simulink library "powerlib_models"  (Simulink 6.0)
settings: Solver=ode45  SolverMode=SingleTasking  StartTime=0.0  StopTime=10.0  RelTol=1e-3
values from neighbouring files (symbols this model uses):
  Ts = get(handles.edit1,'string')    [powergui.m]
undefined symbols (not defined in the file or in its folder): A, a0, a1, a2, a3, a4, a5, Ac, Amplitude, Amplitudes, B, BaseCurrent, BaseFlux, Bc, C, Capacitance, Cc, Columns, ConnectionType, Cs, ctrl, current, Current, damp, Dc, Dd, DiscIntNeverNeededParam, dref, dwo, exc, excAxis, F, Flux, fnom, Frequency, FreqVps, Gain1, gate, GH, GHd, GI, GId, GL, GLd, H, HarmonicGeneration, HT, hyd, I1_init, ib, ib2, Id1o, Inductance, InitialFlux, InitialSlope, io, Iq1o, isfinite, j, J ... (+138)
libraries: powerlib_models x32, powerlib_extras x4
(part 3 of 11)

== system powerlib_models/Continuous/diode (logical) ==
  v : Inport  Port=1  LatchInput=off
  0 {1..4} (4 alike) : Constant  Value=0
  Break Alg. Loop : Subsystem  mask{Nsw=1}
      mask prompts: Nsw "number of switches"
  Constant : Constant  Value=zeros(Nsw,1)
  Data Type  Conversion1 : DataTypeConversion  OutDataTypeMode=boolean  SaturateOnIntegerOverflow=on  RndMeth=Zero
  Data Type  Conversion2 : DataTypeConversion  OutDataTypeMode=boolean  SaturateOnIntegerOverflow=on  RndMeth=Zero
  Data Type  Conversion3 : DataTypeConversion  OutDataTypeMode=boolean  SaturateOnIntegerOverflow=on  RndMeth=Zero
  Gain : Gain  Gain=1./Rsw  SaturateOnIntegerOverflow=on
  Mux : Mux  Inputs=2
  Saturation : Saturate  UpperLimit=inf  LowerLimit=0
  Sum : Sum  Inputs=|++  SaturateOnIntegerOverflow=on  InputSameDT=on
  Switch : Switch  Threshold=0.5  InputSameDT=on
  b5 : RelationalOperator  Operator=>  InputSameDT=on
  b6 : RelationalOperator  Operator=>  InputSameDT=on
  b7 : RelationalOperator  Operator===  InputSameDT=on
  or2 : Logic  Operator=OR
  or3 : Logic
  vf : Constant  Value=Vf
  i : Outport  InitialOutput=0
  status : Outport  Port=2  InitialOutput=0
  m : Outport  Port=3  InitialOutput=0
  Vf : Outport  Port=4  InitialOutput=0
  wires:
  0 3/1 -> b7/2
  0 2/1 -> b6/2
  v/1 -> b6/1, Gain/1, Sum/1  "Diode voltage"
  Mux/1 -> m/1  "measurement signals"
  b6/1 -> Data Type  Conversion2/1  "Voltage > 0"
  or3/1 -> or2/2
  or2/1 -> Break Alg. Loop/1(In1)
  Break Alg. Loop/1(Out1) -> status/1, Switch/2  "status"
  0 4/1 -> b5/2
  b5/1 -> Data Type  Conversion1/1  "Current > 0"
  Constant/1 -> i/1
  Sum/1 -> Mux/2  "V = Vak + Vf"
  vf/1 -> Sum/2, Vf/1
  b7/1 -> Data Type  Conversion3/1  "Current = 0"
  Data Type  Conversion1/1 -> or2/1
  Data Type  Conversion2/1 -> or3/1
  Data Type  Conversion3/1 -> or3/2
  Switch/1 -> Saturation/1
  0 1/1 -> Switch/3
  Saturation/1 -> Mux/1, b7/1, b5/1  "Diode current"
  Gain/1 -> Switch/1  "Diode current"

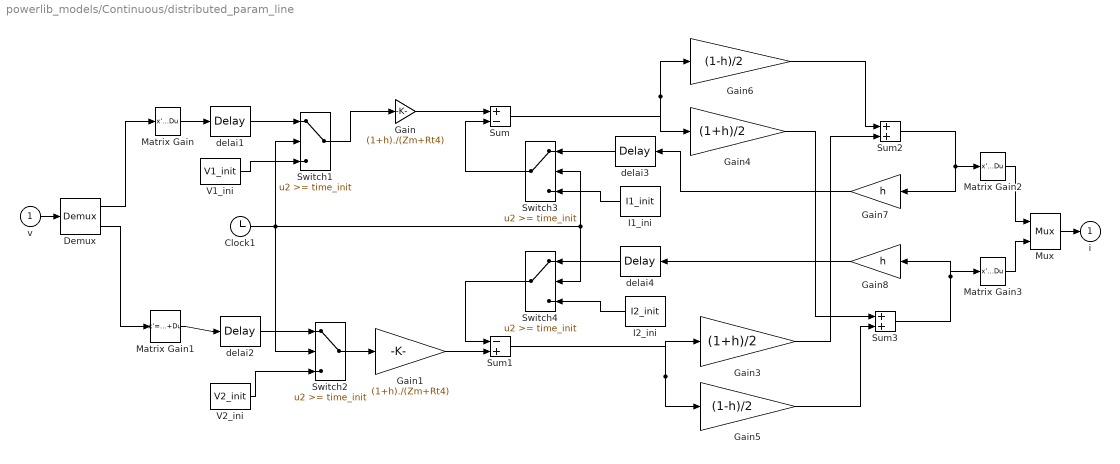
== system powerlib_models/Continuous/distributed_param_line ==
  v : Inport  Port=1  LatchInput=off
  Clock1 : Clock
      settings: Decimation=10
  Demux : Demux  Outputs=[nphase,nphase]
  Gain : Gain  Gain=(1+h)./(Zm+Rt4)  SaturateOnIntegerOverflow=on
  Gain1 : Gain  Gain=(1+h)./(Zm+Rt4)  SaturateOnIntegerOverflow=on
  Gain3 : Gain  Gain=(1+h)/2  SaturateOnIntegerOverflow=on
  Gain4 : Gain  Gain=(1+h)/2  SaturateOnIntegerOverflow=on
  Gain5 : Gain  Gain=(1-h)/2  SaturateOnIntegerOverflow=on
  Gain6 : Gain  Gain=(1-h)/2  SaturateOnIntegerOverflow=on
  Gain7 : Gain  Orientation=left  Gain=h  SaturateOnIntegerOverflow=on
  Gain8 : Gain  Orientation=left  Gain=h  SaturateOnIntegerOverflow=on
  I1_ini : FromWorkspace  Orientation=left  VariableName=I1_init  SampleTime=0
  I2_ini : FromWorkspace  Orientation=left  VariableName=I2_init  SampleTime=0
  Matrix Gain : StateSpace  A=[]  B=[]  C=[]  D=K  mask(Matrix Gain){@1=Ti'}
      mask prompts: @1 "Gain matrix:"
      mask help: Matrix Gain.
      mask init:
      | K = @1;
      mask Help: Multiplies input vector by entered matrix to produce output vector (y=Au).
      mask Display: disp('K')
  Matrix Gain1 : StateSpace  A=[]  B=[]  C=[]  D=K  mask(Matrix Gain){@1=Ti'}
      mask prompts: @1 "Gain matrix:"
      mask help: Matrix Gain.
      mask init:
      | K = @1;
      mask Help: Multiplies input vector by entered matrix to produce output vector (y=Au).
      mask Display: disp('K')
  Matrix Gain2 : StateSpace  A=[]  B=[]  C=[]  D=K  mask(Matrix Gain){@1=Ti}
      mask prompts: @1 "Gain matrix:"
      mask help: Matrix Gain.
      mask init:
      | K = @1;
      mask Help: Multiplies input vector by entered matrix to produce output vector (y=Au).
      mask Display: disp('K')
  Matrix Gain3 : StateSpace  A=[]  B=[]  C=[]  D=K  mask(Matrix Gain){@1=Ti}
      mask prompts: @1 "Gain matrix:"
      mask help: Matrix Gain.
      mask init:
      | K = @1;
      mask Help: Multiplies input vector by entered matrix to produce output vector (y=Au).
      mask Display: disp('K')
  Mux : Mux  Inputs=[nphase,nphase]
  Sum : Sum  Inputs=+-  SaturateOnIntegerOverflow=on  InputSameDT=on
  Sum1 : Sum  Inputs=-+  SaturateOnIntegerOverflow=on  InputSameDT=on
  Sum2 : Sum  SaturateOnIntegerOverflow=on  InputSameDT=on
  Sum3 : Sum  SaturateOnIntegerOverflow=on  InputSameDT=on
  Switch1 : Switch  Threshold=time_init  InputSameDT=on
  Switch2 : Switch  Threshold=time_init  InputSameDT=on
  Switch3 : Switch  Orientation=left  Threshold=time_init  InputSameDT=on
  Switch4 : Switch  Orientation=left  Threshold=time_init  InputSameDT=on
  V1_ini : FromWorkspace  VariableName=V1_init  SampleTime=0
  V2_ini : FromWorkspace  VariableName=V2_init  SampleTime=0
  delai1 : TransportDelay  DelayTime=to
  delai2 : TransportDelay  DelayTime=to
  delai3 : TransportDelay  Orientation=left  DelayTime=to
  delai4 : TransportDelay  Orientation=left  DelayTime=to
  i : Outport  InitialOutput=0
  wires:
  Matrix Gain2/1 -> Mux/1
  Matrix Gain3/1 -> Mux/2
  Demux/2 -> Matrix Gain1/1
  Matrix Gain1/1 -> delai2/1
  Demux/1 -> Matrix Gain/1
  Matrix Gain/1 -> delai1/1
  Gain4/1 -> Sum3/1
  Gain3/1 -> Sum2/2
  Gain6/1 -> Sum2/1
  Gain5/1 -> Sum3/2
  Gain/1 -> Sum/1
  Gain1/1 -> Sum1/2
  v/1 -> Demux/1
  Mux/1 -> i/1
  Sum3/1 -> Gain8/1, Matrix Gain3/1
  Gain7/1 -> delai3/1
  Sum2/1 -> Gain7/1, Matrix Gain2/1
  Gain8/1 -> delai4/1
  delai1/1 -> Switch1/1
  V1_ini/1 -> Switch1/3
  Switch2/1 -> Gain1/1
  Switch1/1 -> Gain/1
  delai2/1 -> Switch2/1
  V2_ini/1 -> Switch2/3
  Sum/1 -> Gain4/1, Gain6/1
  Sum1/1 -> Gain3/1, Gain5/1
  delai3/1 -> Switch3/1
  Switch3/1 -> Sum/2
  Switch4/1 -> Sum1/1
  delai4/1 -> Switch4/1
  Clock1/1 -> Switch4/2, Switch3/2, Switch2/2, Switch1/2
  I1_ini/1 -> Switch3/3
  I2_ini/1 -> Switch4/3

== system powerlib_models/Continuous/hysteresis_transformer ==
  v : Inport  Port=1  LatchInput=off
  Hysteresis ( always SI ) : Subsystem
  fluxinit : Integrator  InitialCondition=InitialFlux
  i : Outport  InitialOutput=0
  f : Outport  Port=2  InitialOutput=0
  wires:
  Hysteresis ( always SI )/1(Out1) -> i/1
  v/1 -> fluxinit/1
  fluxinit/1 -> Hysteresis ( always SI )/1(In1), f/1  "flux displayed by Multimeter block"

== system powerlib_models/Continuous/ideal_switch ==
  v : Inport  Port=1  LatchInput=off
  g : Inport  Port=2  LatchInput=off
  0 1 : Constant  Value=0
  1/Rsw : Gain  Gain=1./Rsw  SaturateOnIntegerOverflow=on
  Constant : Constant  Value=zeros(Nsw,1)
  Data Type Conversion : DataTypeConversion  OutDataTypeMode=double  SaturateOnIntegerOverflow=on  RndMeth=Zero
  Mux : Mux  Inputs=2
  Switch : Switch  Threshold=0.5  InputSameDT=on
  i : Outport  InitialOutput=0
  Status : Outport  Port=2  InitialOutput=0
  m : Outport  Port=3  InitialOutput=0
  wires:
  g/1 -> Switch/2, Data Type Conversion/1
  Mux/1 -> m/1  "measurement signals"
  v/1 -> Mux/2, 1/Rsw/1  "Vak"
  Constant/1 -> i/1
  1/Rsw/1 -> Switch/1  "Iak"
  Switch/1 -> Mux/1
  0 1/1 -> Switch/3
  Data Type Conversion/1 -> Status/1

== system powerlib_models/Continuous/saturable_transformer ==
  v : Inport  Port=1  LatchInput=off
  Integrator : Integrator  InitialCondition=InitialFlux
  Look-Up Table : Lookup  DialogController=Simulink.DDGSource  InputValues=SaturationFlux  OutputValues=SaturationCurrent  SaturateOnIntegerOverflow=on
  i : Outport  InitialOutput=0
  f : Outport  Port=2  InitialOutput=0
  wires:
  Look-Up Table/1 -> i/1
  v/1 -> Integrator/1
  Integrator/1 -> Look-Up Table/1, f/1  "flux"

== system powerlib_models/Continuous/simplified_sync_mach ==
  v : Inport  Port=1  LatchInput=off
  e : Inport  Port=2  LatchInput=off
  theta_e : Inport  Port=3  LatchInput=off
  wm : Inport  Port=4  LatchInput=off
  1\p : Gain  Gain=1/p  SaturateOnIntegerOverflow=on
  Selector : Selector  Elements=sel  InputPortWidth=3
  Subsystem : Subsystem
  Vt : Subsystem
  Z : Subsystem
      mask Display: disp('Z')
  gen : Subsystem
      mask Display: disp('gen')
  ib : Gain  Gain=ib  SaturateOnIntegerOverflow=on
  wattmeter : Subsystem  Orientation=left
      mask Display: disp('wattmeter')
  i : Outport  InitialOutput=0
  m : Outport  Port=2  InitialOutput=0
  Pe : Outport  Orientation=left  Port=3  InitialOutput=0
  wires:
  Selector/1 -> i/1
  ib/1 -> Selector/1
  wattmeter/1(Pe) -> Subsystem/6(Pe), Pe/1
  e/1 -> gen/2(E)
  theta_e/1 -> 1\p/1, gen/1(theta)
  v/1 -> Vt/1(V)
  1\p/1 -> Subsystem/4(theta)
  wm/1 -> Subsystem/5(wm)
  Z/1(i) -> ib/1, Subsystem/1(i), wattmeter/1(i)
  gen/1(e) -> Subsystem/3(e), Z/1(e), wattmeter/2(v)  "e"
  Vt/1(Vn) -> gen/3(Vn)
  Vt/2(Vabc) -> Z/2(v), Subsystem/2(v)
  Subsystem/1(*) -> m/1

== system powerlib_models/Continuous/surge_arrester ==
  v : Inport  Port=1  LatchInput=off
  Abs : Abs  SaturateOnIntegerOverflow=on
  Break Alg. Loop : TransferFcn  Denominator="[BreakLoop*0.01e-6  1]"
  Product : Product  SaturateOnIntegerOverflow=on  InputSameDT=on
  Sign : Signum  Orientation=down
  Switch1 : Switch  Threshold=ic1  InputSameDT=on
  Switch2 : Switch  Threshold=ic2  InputSameDT=on
  segment1 : Fcn  Expr=p1*(u/uref)^a1
  segment2 : Fcn  Expr=p2*(u/uref)^a2
  segment3 : Fcn  Expr=p3*(u/uref)^a3
  I : Outport  InitialOutput=0
  wires:
  Sign/1 -> Product/2
  Abs/1 -> segment1/1, segment2/1, segment3/1
  segment1/1 -> Switch1/3, Switch1/2
  segment2/1 -> Switch1/1
  Switch2/1 -> Product/1
  Switch1/1 -> Switch2/2, Switch2/3
  segment3/1 -> Switch2/1
  v/1 -> Break Alg. Loop/1
  Break Alg. Loop/1 -> Sign/1, Abs/1
  Product/1 -> I/1

== system powerlib_models/Continuous/synchronous_machine ==
  v : Inport  Port=1  PortDimensions=2  LatchInput=off
  vf : Inport  Port=2  PortDimensions=1  LatchInput=off
  theta_e : Inport  Port=3  PortDimensions=1  LatchInput=off
  we : Inport  Port=4  PortDimensions=1  LatchInput=off
  Delta angle : Subsystem
  Mux : Mux  Inputs=[3,10,1,1,1]
  Mux1 : Mux  Inputs=[ 1 1 2 ]
  PQ : Subsystem
  Subsystem : Subsystem
  Te electrical torque : Fcn  Expr=u[1]*u[3]-u[2]*u[4]
  abc2qd : Subsystem
  currents and mutual fluxes : Subsystem
      mask Display: disp('currents\nand\nmutual\nfluxes')
  ia,ib : Selector  Elements=1:2  InputPortWidth=3
  phid : Subsystem
      mask Display: disp('phid')
  phifd : Subsystem
      mask Display: disp('phifd')
  phikd : Subsystem
      mask Display: disp('phikd')
  phikq1 : Subsystem
      mask Display: disp('phikq1')
  phikq2 : Subsystem
      mask Display: disp('phikq2')
  phiq : Subsystem
      mask Display: disp('phiq')
  qd2abc : Subsystem
  vkd : Ground
  vkq2 : Ground
  i : Outport  InitialOutput=0
  m : Outport  Port=2  InitialOutput=0
  Te : Outport  Port=3  InitialOutput=0
  wires:
  vf/1 -> Subsystem/1(Vf)
  currents and mutual fluxes/2("iq,id,ifd, ikq1,ikq2,ikd, phimq,phimd,vq,vd") -> Mux/2
  vkq2/1 -> phikq2/1(vkq2)
  abc2qd/2(vq) -> phiq/1(vq), Delta angle/1(Vq), currents and mutual fluxes/7(vq), PQ/1(Vq)
  vkd/1 -> phikd/2(vkd)
  phiq/1(phiq) -> phid/2(phiq), currents and mutual fluxes/1(phiq), Mux1/2  "phi_q"
  qd2abc/1(is(A)) -> ia,ib/1  "iabc"
  currents and mutual fluxes/1(phimq) -> phiq/4(phimq), phikq2/2(phimq), phikq1/1(phimq)
  qd2abc/2(is(pu)) -> Mux/1
  abc2qd/1(cos,sin) -> qd2abc/1(sin,cos)
  currents and mutual fluxes/3(iq,id) -> PQ/3(Iq), qd2abc/2(iq,id), Mux1/3  "iq,id"
  ia,ib/1 -> i/1
  phid/1(phid) -> phiq/3(phid), currents and mutual fluxes/3(phid), Mux1/1  "phi_d"
  abc2qd/3(vd) -> phid/3(vd), Delta angle/2(Vd), currents and mutual fluxes/8(vd), PQ/2(Vd)
  v/1 -> abc2qd/1(v)
  phikd/1(phikd) -> currents and mutual fluxes/6(phikd)
  phifd/1(phifd) -> currents and mutual fluxes/4(phifd)
  phikq1/1(phikq1) -> currents and mutual fluxes/5(phikq1)
  phikq2/1(phikq2) -> currents and mutual fluxes/2(phikq2)
  Subsystem/1(Vkq1) -> phikq1/2(vkq1)
  Subsystem/2(Vfd) -> phifd/1(vfd)
  Mux/1 -> m/1
  currents and mutual fluxes/4(phimd) -> phid/4(phimd), phifd/2(phimd), phikd/1(phimd)
  PQ/1(Peo) -> Mux/4
  PQ/2(Qeo) -> Mux/5
  Delta angle/1(delta) -> Mux/3
  theta_e/1 -> abc2qd/2(theta)
  we/1 -> phid/1(w), phiq/2(w)
  Mux1/1 -> Te electrical torque/1
  Te electrical torque/1 -> Te/1

== system powerlib_models/Continuous/thyristor (logical) ==
  v : Inport  Port=1  LatchInput=off
  g : Inport  Port=2  LatchInput=off
  0 {1..4} (4 alike) : Constant  Value=0
  1/Rsw : Gain  Orientation=down  Gain=1./Rsw  SaturateOnIntegerOverflow=on
  Break Alg. Loop : Subsystem  mask{Nsw=1}
      mask prompts: Nsw "number of switches"
  Constant : Constant  Value=zeros(Nsw,1)
  Data Type  Conversion{1..4} (4 alike) : DataTypeConversion  OutDataTypeMode=boolean  SaturateOnIntegerOverflow=on  RndMeth=Zero
  Mux : Mux  Inputs=2
  Saturation : Saturate  UpperLimit=inf  LowerLimit=0
  Sum : Sum  Inputs=|++  SaturateOnIntegerOverflow=on  InputSameDT=on
  Switch : Switch  Threshold=0.5  InputSameDT=on
  b5 : RelationalOperator  Operator=>  InputSameDT=on
  b6 : RelationalOperator  Operator=>  InputSameDT=on
  b7 : RelationalOperator  Operator===  InputSameDT=on
  or2 : Logic  Operator=OR
  or3 : Logic  Inputs=3
  vf : Constant  Value=Vf
  i : Outport  InitialOutput=0
  Status : Outport  Port=2  InitialOutput=0
  m : Outport  Port=3  InitialOutput=0
  Vf : Outport  Port=4  InitialOutput=0
  wires:
  Data Type  Conversion4/1 -> or3/3
  Data Type  Conversion3/1 -> or3/2
  g/1 -> Data Type  Conversion4/1  "gate signal"
  0 2/1 -> b6/2
  or3/1 -> or2/2  "Gate = 1 Voltage > 0 Current = 0"
  Mux/1 -> m/1  "measurement signals"
  0 3/1 -> b7/2
  b7/1 -> Data Type  Conversion3/1  "Current = 0"
  or2/1 -> Break Alg. Loop/1(In1)
  Break Alg. Loop/1(Out1) -> Status/1, Switch/2
  0 1/1 -> b5/2
  Constant/1 -> i/1
  v/1 -> b6/1, Sum/1, 1/Rsw/1  "Vak"
  Sum/1 -> Mux/2
  vf/1 -> Sum/2, Vf/1
  b5/1 -> Data Type  Conversion1/1  "Current > 0"
  Data Type  Conversion1/1 -> or2/1
  b6/1 -> Data Type  Conversion2/1  "Voltage > 0"
  Data Type  Conversion2/1 -> or3/1
  Switch/1 -> Saturation/1
  0 4/1 -> Switch/3
  Saturation/1 -> Mux/1, b7/1, b5/1
  1/Rsw/1 -> Switch/1  "Iak"

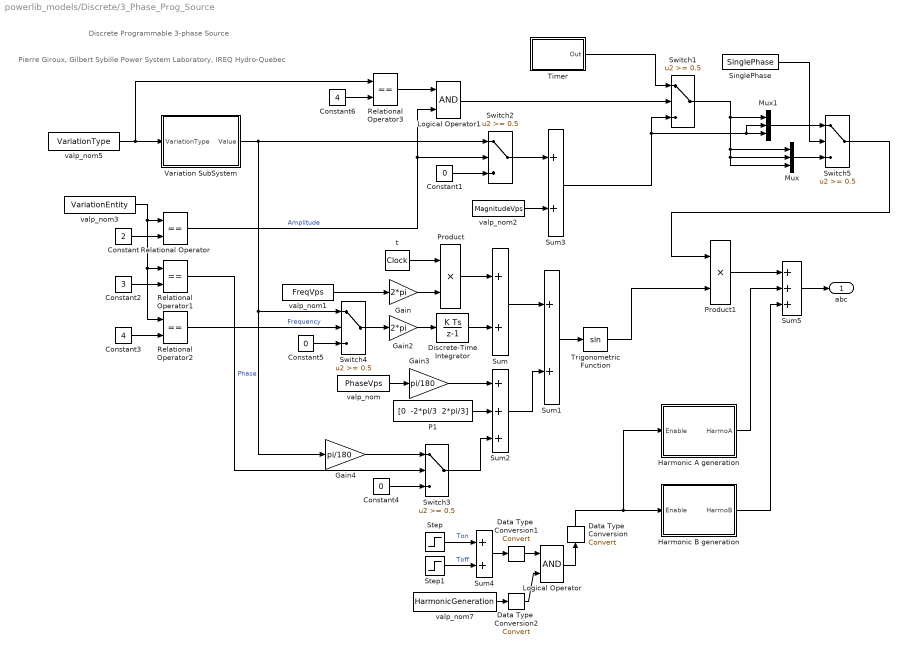
== system powerlib_models/Discrete/3_Phase_Prog_Source ==
  note: Pierre Giroux, Gilbert Sybille
      | Power System Laboratory, IREQ
      | Hydro-Quebec
  note: Discrete Programmable 3-phase Source
  Constant : Constant  Value=2
  Constant1 : Constant  Value=0
  Constant2 : Constant  Value=3
  Constant3 : Constant  Value=4
  Constant4 : Constant  Value=0
  Constant5 : Constant  Value=0
  Constant6 : Constant  Value=4
  Data Type  Conversion : DataTypeConversion  Orientation=up  OutDataTypeMode=double  SaturateOnIntegerOverflow=on  RndMeth=Zero
  Data Type  Conversion1 : DataTypeConversion  OutDataTypeMode=boolean  SaturateOnIntegerOverflow=on  RndMeth=Zero
  Data Type  Conversion2 : DataTypeConversion  OutDataTypeMode=boolean  SaturateOnIntegerOverflow=on  RndMeth=Zero
  Discrete-Time Integrator : DiscreteIntegrator  SampleTime=Ts  ICPrevOutput=DiscIntNeverNeededParam  ICPrevScaledInput=DiscIntNeverNeededParam
  Gain : Gain  Gain=2*pi  SaturateOnIntegerOverflow=on
  Gain2 : Gain  Gain=2*pi  SaturateOnIntegerOverflow=on
  Gain3 : Gain  Gain=pi/180  SaturateOnIntegerOverflow=on
  Gain4 : Gain  Gain=pi/180  SaturateOnIntegerOverflow=on
  Harmonic A generation : Subsystem  mask(Harmonic generation){Freq_Vps=FreqVps, n_Harmo=n_HarmoA, Mag_Harmo=Mag_HarmoA, Phase_Harmo=Phase_HarmoA, Seq_Harmo=Seq_HarmoA, Ts=Ts}
      mask prompts: Ts "Sample time:"
  Harmonic B generation : Subsystem  mask(Harmonic generation){Freq_Vps=FreqVps, n_Harmo=n_HarmoB, Mag_Harmo=Mag_HarmoB, Phase_Harmo=Phase_HarmoB, Seq_Harmo=Seq_HarmoB, Ts=Ts}
      mask prompts: Ts "Sample time:"
  Logical Operator : Logic
  Logical Operator1 : Logic
  Mux : Mux  Inputs=3
  Mux1 : Mux  Inputs=3
  P1 : Constant  Value="[0  -2*pi/3  2*pi/3]"
  Product : Product  SaturateOnIntegerOverflow=on  InputSameDT=on
  Product1 : Product  SaturateOnIntegerOverflow=on  InputSameDT=on
  Relational Operator{,1..3} (4 alike) : RelationalOperator  Operator===  InputSameDT=on
  SinglePhase : Constant  Value=SinglePhase
  Step : Step  Time=Ton_Harmo  SampleTime=Ts
  Step1 : Step  Time=Toff_Harmo  After=-1  SampleTime=Ts
  Sum{,1,3..4} (4 alike) : Sum  SaturateOnIntegerOverflow=on  InputSameDT=on
  Sum2 : Sum  Inputs=+++  SaturateOnIntegerOverflow=on  InputSameDT=on
  Sum5 : Sum  Inputs=+++  SaturateOnIntegerOverflow=on  InputSameDT=on
  Switch{1..5} (5 alike) : Switch  Threshold=0.5  InputSameDT=on
  Timer : Subsystem  mask(Timer){t=TimeValues, e=Amplitudes, Ts=Ts}
      mask prompts: t "Time (s):"; e "Amplitude:"; Ts "Sample time (s)"
      mask help:
      | Generates a signal changing  at specified times.
      |
      | Value of the signal at time zero must  be specified.
      mask init: same as powerlib_models/Continuous/3_Phase_Prog_Source/Timer
      mask Display: plot( tv(2:end-1), opv(2:end-1) )
  Trigonometric Function : Trigonometry
  Variation SubSystem : Subsystem  mask(Variation Subsystem){VariationStep=VariationStep, VariationRate=VariationRate, VariationFreq=VariationFrequency, VariationMag=VariationMagnitude, Ton_Variation=Ton_Variation, Toff_Variation=Toff_Variation, Ts=Ts}
      mask prompts: Ts "Sample time:"
  t : DigitalClock  SampleTime=Ts
  valp_nom : Constant  Value=PhaseVps
  valp_nom1 : Constant  Value=FreqVps
  valp_nom2 : Constant  Value=MagnitudeVps
  valp_nom3 : Constant  Value=VariationEntity
  valp_nom5 : Constant  Value=VariationType
  valp_nom7 : Constant  Value=HarmonicGeneration
  abc : Outport  InitialOutput=0
  wires:
  Logical Operator1/1 -> Switch1/2
  Relational Operator3/1 -> Logical Operator1/1
  Switch5/1 -> Product1/1
  Switch1/1 -> Mux1/1, Mux/3, Mux/2, Mux/1
  Mux/1 -> Switch5/3
  SinglePhase/1 -> Switch5/2
  Mux1/1 -> Switch5/1
  Timer/1(Out) -> Switch1/1
  Sum3/1 -> Mux1/2, Mux1/3, Switch1/3
  Constant6/1 -> Relational Operator3/2
  Gain4/1 -> Switch3/1
  Harmonic B generation/1(HarmoB) -> Sum5/3
  Step1/1 -> Sum4/2  "Toff"
  Step/1 -> Sum4/1  "Ton"
  Sum5/1 -> abc/1
  Harmonic A generation/1(HarmoA) -> Sum5/2
  Constant5/1 -> Switch4/3
  Constant3/1 -> Relational Operator2/2
  Constant2/1 -> Relational Operator1/2
  valp_nom3/1 -> Relational Operator1/1, Relational Operator2/1, Relational Operator/1
  Constant/1 -> Relational Operator/2
  Relational Operator2/1 -> Switch4/2  "Frequency"
  Switch4/1 -> Gain2/1
  Variation SubSystem/1(Value) -> Gain4/1, Switch4/1, Switch2/1
  Relational Operator1/1 -> Switch3/2  "Phase"
  Constant4/1 -> Switch3/3
  Switch3/1 -> Sum2/3
  valp_nom5/1 -> Relational Operator3/1, Variation SubSystem/1(VariationType)
  Relational Operator/1 -> Logical Operator1/2, Switch2/2  "Amplitude"
  valp_nom2/1 -> Sum3/2
  Sum2/1 -> Sum1/2
  Constant1/1 -> Switch2/3
  Switch2/1 -> Sum3/1
  Product1/1 -> Sum5/1
  valp_nom1/1 -> Gain/1
  valp_nom/1 -> Gain3/1
  Gain3/1 -> Sum2/1
  Trigonometric Function/1 -> Product1/2
  P1/1 -> Sum2/2
  Discrete-Time Integrator/1 -> Sum/2
  Gain2/1 -> Discrete-Time Integrator/1
  Sum1/1 -> Trigonometric Function/1
  Sum/1 -> Sum1/1
  t/1 -> Product/1
  Gain/1 -> Product/2
  Product/1 -> Sum/1
  Logical Operator/1 -> Data Type  Conversion/1
  Data Type  Conversion/1 -> Harmonic A generation/1(Enable), Harmonic B generation/1(Enable)
  Sum4/1 -> Data Type  Conversion1/1
  Data Type  Conversion1/1 -> Logical Operator/1
  valp_nom7/1 -> Data Type  Conversion2/1
  Data Type  Conversion2/1 -> Logical Operator/2

== system powerlib_models/Discrete/ASM_mechanics ==
  Tm : Inport  Port=1  LatchInput=off
  Te : Inport  Port=2  LatchInput=off
  1\p : Gain  Gain=1/p  SaturateOnIntegerOverflow=on
  1\p1 : Gain  Gain=[Nb2;Tb2;1]  SaturateOnIntegerOverflow=on
  1_2H : Gain  Gain=1/(2*H)  SaturateOnIntegerOverflow=on
  1_Tb2 : Gain  Gain=1/Tb2  SaturateOnIntegerOverflow=on
  Discrete-Time Integrator : DiscreteIntegrator  InitialCondition=wmo  SampleTime=Ts  ICPrevOutput=DiscIntNeverNeededParam  ICPrevScaledInput=DiscIntNeverNeededParam
  Discrete-Time Integrator1 : DiscreteIntegrator  InitialCondition=tho  SampleTime=Ts  ICPrevOutput=DiscIntNeverNeededParam  ICPrevScaledInput=DiscIntNeverNeededParam
  F : Gain  Orientation=left  Gain=F  SaturateOnIntegerOverflow=on
  Mux3 : Mux  Inputs=2
  Mux4 : Mux  Inputs=3
  Sum : Sum  Inputs=-+-  SaturateOnIntegerOverflow=on  InputSameDT=on
  web_psb : Gain  Gain=web_psb  SaturateOnIntegerOverflow=on
  m : Outport
  thr,wr : Outport  Port=2
  wires:
  Mux4/1 -> 1\p1/1
  Mux3/1 -> thr,wr/1
  Tm/1 -> 1_Tb2/1
  Sum/1 -> 1_2H/1
  1_2H/1 -> Discrete-Time Integrator/1
  Discrete-Time Integrator/1 -> F/1, Mux3/2, Mux4/1, web_psb/1
  F/1 -> Sum/3
  1_Tb2/1 -> Sum/1
  Te/1 -> Mux4/2, Sum/2
  web_psb/1 -> Discrete-Time Integrator1/1
  1\p/1 -> Mux4/3
  Discrete-Time Integrator1/1 -> 1\p/1, Mux3/1
  1\p1/1 -> m/1  "w,Te,thr"

== system powerlib_models/Discrete/Dynamic_Load ==
  v : Inport  Port=1  PortDimensions=2  LatchInput=off
  PQ : Inport  Port=2  PortDimensions=2  LatchInput=off
  Complex to Real-Imag : ComplexToRealImag  Orientation=left
  Demux : Demux  Outputs=2
  Discrete 3-phase PLL : Subsystem  mask(Discrete 3-phase PLL){Par_Init=[Pha_V0  fnom], ParK=[60 1400], Ts=Ts}
      mask prompts: Par_Init "Initial inputs:[ Phase(degrees)   Frequency(Hz) ]"; ParK "Regulator gains [ Kp  Ki ]"; Ts "Sample time:"
      mask init:
      | Kp=ParK(1);
      | Ki=ParK(2);
      | Phase_Init=Par_Init(1);
      | Finit=Par_Init(2);
  Discrete Variable Frequency Mean value : powerlib_extras/Discrete Measurements/Discrete Variable Frequency Mean value  Finit=fnom  Fmin=45  Vinit=Mag_V0  Ts=Ts
  Discrete Variable Frequency Mean value1 : powerlib_extras/Discrete Measurements/Discrete Variable Frequency Mean value  Finit=fnom  Fmin=45  Vinit=0  Ts=Ts
  Ground : Ground  Orientation=left
  Mux1 : Mux  Orientation=left  Inputs=3
  Positive Sequence  current : Subsystem
  Real-Imag to Complex : RealImagToComplex
  Real-Imag to Complex1 : RealImagToComplex
  Selector : Selector  Orientation=left  Elements=1:2  InputPortWidth=3
  Unit Delay2 : UnitDelay  Orientation=left  X0=I1_init*exp(-j*Pha_V0*pi/180)  SampleTime=Ts
  V> pu : Gain  Gain=1/Vbase  SaturateOnIntegerOverflow=on
  dq0_to_abc Transformation : powerlib_extras/Measurements/dq0_to_abc Transformation  Orientation=left
  i : Outport  Orientation=left
  m : Outport  Port=2
  wires:
  dq0_to_abc Transformation/1 -> Selector/1
  Selector/1 -> i/1
  v/1 -> V> pu/1
  V> pu/1 -> Discrete 3-phase PLL/1(Vab_bc (pu))
  Real-Imag to Complex/1 -> Positive Sequence  current/1(V1(pu))
  Mux1/1 -> dq0_to_abc Transformation/1
  Unit Delay2/1 -> Complex to Real-Imag/1
  Discrete 3-phase PLL/3(Vq) -> Discrete Variable Frequency Mean value1/2
  Ground/1 -> Mux1/3
  Discrete Variable Frequency Mean value/1 -> Real-Imag to Complex/1
  Discrete Variable Frequency Mean value1/1 -> Real-Imag to Complex/2
  Positive Sequence  current/1(I1(A)) -> Unit Delay2/1
  Complex to Real-Imag/1 -> Mux1/1
  Complex to Real-Imag/2 -> Mux1/2
  Discrete 3-phase PLL/2(Vd) -> Discrete Variable Frequency Mean value/2
  Discrete 3-phase PLL/4(sin_cos) -> dq0_to_abc Transformation/2
  Discrete 3-phase PLL/1(Freq) -> Discrete Variable Frequency Mean value/1, Discrete Variable Frequency Mean value1/1
  PQ/1 -> Demux/1
  Demux/1 -> Real-Imag to Complex1/1
  Demux/2 -> Real-Imag to Complex1/2
  Real-Imag to Complex1/1 -> Positive Sequence  current/2(S_ext)
  Positive Sequence  current/2(VPQ) -> m/1

== system powerlib_models/Discrete/Excitation_System ==
  note: link disabled
  note: link disabled
  vref : Inport  Port=1  LatchInput=off
  vd : Inport  Port=2  LatchInput=off
  vq : Inport  Port=3  LatchInput=off
  vstab : Inport  Port=4  LatchInput=off
  Damping kf.s / (tf.s +1) : Subsystem  Orientation=left
  Exciter  1 / (te.s + ke) : Subsystem
  Lead Lag Compensator tc.s+1 / tb.s+1 : Subsystem  AncestorBlock=|  mask(Discrete Lead-Lag Controller){T1=tc, T2=tb, V_Init=ke*v0(2)/ka, Ts=Ts}
      | powerlib_extras/Discrete 
      | Control Blocks/Discrete
      | Lead-Lag
      mask prompts: T1 "Time constant T1 (s):"; T2 "Time constant T2 (s):"; V_Init "Initial input and output:"; Ts "Sample time (s):"
      mask help:
      | This block implements a discrete lead-lag controller:
      |
      |          1+T1s
      | H(s)= ------
      |          1+T2s
      |
      | States are initialized according to initial input anf output value so that simulation starts in steady state.
      mask init:
      | numc=[T1 1];
      | denc=[T2 1];
      | [Ac,Bc,Cc,Dc]=tf2ss(numc,denc);
      | 
      | %  Conversion to discrete transfer function
      | nstates = size(Ac,1);
      | invexp = inv(eye(nstates) - (Ts/2)*Ac);
      | Ad = invexp*(eye(nstates) + (Ts/2)*Ac);
      | Bd = invexp*Bc;
      | Cd = Cc*invexp*Ts;
      | Dd = Cc*invexp*Bc*(Ts/2) + Dc;
      | %
      | % Compute Initial states
      | I=eye(size(Ac));
      | x0c=inv(-Ac)*Bc*V_Init;
      | x0d=(I-Ac*Ts/2)*x0c/Ts - Bc/2*V_Init;
      | 
      | if T1==0 & T2==0, Dd=1; end
      mask Display: disp('1+T1s\n---\n1+T2s')
  Low Pass Filter 1 / (tr.s +1) (with IC) : Subsystem  AncestorBlock=|  mask(Discrete 1st-Order Filter){FilterType=Lowpass, Tc=tr, Ts=Ts, Initialize=on, Vac_Init=[0 0 60], Vdc_Init=v0(1), PlotResponse=off, param1=[1 500 0.1]}
      | powerlib_extras/Discrete 
      | Control Blocks/Discrete
      | 1st-Order
      | Discrete Filter
      mask prompts: FilterType "Filter Type:"; Tc "Time constant (s):"; Ts "Sample time:"; Initialize "Initialize filter states"; Vac_Init "AC initial input: [ Mag  Phase(degrees)  Freq(Hz) ]"; Vdc_Init "DC Initial input:"; PlotResponse "Plot filter response"; param1 "Frequency range(Hz) : [Start  End  Inc.]"
      mask init:
      | switch FilterType
      | case 1, % Lowpass
      |     X=[0 1 2 3 4];
      |     Y=[-2 -2 -3 -4 -4];
      |     numc=1;
      |     denc=[Tc 1];
      | case 2,   % Highpass
      |     X=[0 1 2 3 4];
      |     Y=[-4 -4 -3 -2 -2];
      |     numc=[1 0];
      |     denc=[1 1/Tc];
      | end
      | %
      | [Ac,Bc,Cc,Dc]=tf2ss(numc,denc);
      | %
      | %  Conversion to discrete transfer function
      | nstates = size(Ac,1);
      | invexp = inv(eye(nstates) - (Ts/2)*Ac);
      | Ad = invexp*(eye(nstates) + (Ts/2)*Ac);
      | Bd = invexp*Bc;
      | Cd = Cc*invexp*Ts;
      | Dd = Cc*invexp*Bc*(Ts/2) + Dc;
      | %
      | if Initialize==1  % Compute initial conditions on states
      |     u1=Vac_Init(1)*exp(j*Vac_Init(2)*pi/180);
      |     u2=Vdc_Init*exp(j*90*pi/180);
      |     u=u1+u2;
      |     u0=imag(u); % input at  t=0;
      |     I=eye(size(Ac));
      |     sI1=I*j*(2*pi*Vac_Init(3));
      |     sI2=I*j*0;
      |     x=inv(sI1-Ac)*Bc*u1 + inv(sI2-Ac)*Bc*u2;
      |     x0c=imag(x);
      |     x0d=(I-Ac*Ts/2)*x0c/Ts - Bc/2*u0;
      | else
      |     x0d=0;
      | end
      | 
      | %
      | if PlotResponse==1 % Plot frequency and step response
      |     figure(1)
      |     sys=ss(Ad,Bd,Cd,Dd,Ts);
      |     f=param1(1):param1(3):param1(2);
      |     w=2*pi*f;
      |     [mag phase]=bode(sys,w);
      |     subplot(2,1,1)
      |     plot(f,squeeze(mag))
      |     title('Magnitude')
      |     grid
      |     subplot(2,1,2)
      |     plot(f,squeeze(phase))
      |     title('Phase (degrees)')
      |     xlabel('Hz')
      |     grid
      |     figure(2)
      |     step(sys)
      | end
      mask StyleString: popup(Lowpass|Highpass),edit,edit,checkbox,edit,edit,checkbox,edit
      mask CallbackString: |||p4=get_param(gcb,'Initialize');if strcmp(p4,'on');visible={'on','on','on','on','on','on','on',get_param(gcb,'PlotResponse')};else;visible={'on','on','on','on','off','off','on',get_param(gcb,'PlotResponse')};end;set_param(gcb,'MaskVisibilities',visible)|||p7=get_param(gcb,'PlotResponse');if strcmp(p7,'on');visible={'on','on','on','on',get_param(gcb,'Initialize'),get_param(gcb,'Initialize'),'on','on'};else;visible={'on','on','on','on',get_param(gcb,'Initialize'),get_param(gcb,'Initialize'),'on','off'};end;set_param(gcb,'MaskVisibilities',visible)|
      mask Display: plot(X,Y);
  Main Regulator ka / (ta.s +1) : Subsystem
  Mux : Mux  Inputs=2
  Positive Sequence Voltage : Fcn  Expr=sqrt(u(1)^2 + u(2)^2)
  Sum : Sum  Inputs=++-+-  SaturateOnIntegerOverflow=on  InputSameDT=on
  Unit Delay1 : UnitDelay  Orientation=left  SampleTime=Ts
  Unit Delay2 : UnitDelay  X0=v0(2)  SampleTime=Ts
  Vf0 / ka : Constant  Value=v0(2)/ka
  proportionnal saturation : Subsystem
  Vf : Outport  InitialOutput=0
  wires:
  Unit Delay2/1 -> Vf/1
  Unit Delay1/1 -> Sum/5
  proportionnal saturation/1(Ef) -> Exciter  1 / (te.s + ke)/1(In)
  Lead Lag Compensator tc.s+1 / tb.s+1/1(Out1) -> Main Regulator ka / (ta.s +1)/1(In)
  Sum/1 -> Lead Lag Compensator tc.s+1 / tb.s+1/1(In1)
  Positive Sequence Voltage/1 -> Low Pass Filter 1 / (tr.s +1) (with IC)/1(In)
  vq/1 -> Mux/2
  vd/1 -> Mux/1
  Mux/1 -> Positive Sequence Voltage/1
  vref/1 -> Sum/1
  vstab/1 -> Sum/4
  Low Pass Filter 1 / (tr.s +1) (with IC)/1(Out) -> proportionnal saturation/2(Vtf), Sum/3
  Vf0 / ka/1 -> Sum/2
  Main Regulator ka / (ta.s +1)/1(Out) -> proportionnal saturation/1(Efd)
  Damping kf.s / (tf.s +1)/1(Out) -> Unit Delay1/1
  Exciter  1 / (te.s + ke)/1(Out) -> Unit Delay2/1, Damping kf.s / (tf.s +1)/1(In)

== system powerlib_models/Discrete/GTO-IGBT Bridge ==
  note: *
      | *
      | ||
      | ||
      | *
      | *
      | *
      | ||
      | ||
      | *
      | *
  note: 1
  note: 2
  note: +
  note: -
  note: *
      | *
      | ||
      | ||
      | *
      | *
      | *
      | ||
      | ||
      | *
      | *
  note: 3
  note: 4
  note: ***********************************************
  note: Vcc
  note: A
  note: B
  note: *
      | *
      | ||
      | ||
      | *
      | *
      | *
      | ||
      | ||
      | *
      | *
  note: C
  note: ***********************************************
  note: 5
  note: 6
  note: GTO:
      |  tail current can be turned off by specifying Tf=0 and Tt=0
  note: Diode Logic :
      | 1) Diodes are blocked when complementary GTOs are switched on
      | 2) When no snubber capacitances are used (Cs=inf), diodes are triggered
      | when complementary GTOs are swithed off
  v : Inport  Port=1  LatchInput=off
  g : Inport  Port=2  LatchInput=off
  1/Rsw : Gain  Orientation=up  Gain=1./Rsw  SaturateOnIntegerOverflow=on
  2 : Constant  Value=Tf>0 | Tt>0
  Constant1 : Constant  Value=0
  Data Type  Conversion2 : DataTypeConversion  OutDataTypeMode=double  SaturateOnIntegerOverflow=on  RndMeth=Zero
  Data Type  Conversion3 : DataTypeConversion  OutDataTypeMode=double  SaturateOnIntegerOverflow=on  RndMeth=Zero
  Data Type  Conversion4 : DataTypeConversion  OutDataTypeMode=boolean  SaturateOnIntegerOverflow=on  RndMeth=Zero
  Data Type  Conversion5 : DataTypeConversion  OutDataTypeMode=boolean  SaturateOnIntegerOverflow=on  RndMeth=Zero
  Diode Logic : Subsystem
  GTO Logic : Subsystem
  G_D : Logic  Operator=OR
  Gain : Gain  Orientation=up  Gain=-1  SaturateOnIntegerOverflow=on
  Product : Product  SaturateOnIntegerOverflow=on  InputSameDT=on
  Relational Operator : RelationalOperator  InputSameDT=on
  Tail discrete : Subsystem  TreatAsAtomicUnit=on  mask(Gto tail current){}
  Unit Delay : UnitDelay  SampleTime=Ts
  Unit Delay3 : UnitDelay  SampleTime=Ts
  "Vf " : Subsystem
  iTail : Outport
  status : Outport  Port=2
  Vf : Outport  Port=3
  wires:
  2/1 -> Tail discrete/Enable
  Relational Operator/1 -> Diode Logic/2(Ipos), Data Type  Conversion3/1
  Constant1/1 -> Relational Operator/2
  Unit Delay/1 -> Tail discrete/1(Iak)
  Gain/1 -> Diode Logic/1(Vak)
  Product/1 -> Unit Delay/1  "IGTO"
  Tail discrete/1(itail) -> iTail/1
  1/Rsw/1 -> Product/2, Relational Operator/1
  v/1 -> Gain/1, GTO Logic/1(Vak), 1/Rsw/1
  "Vf "/1(Vf) -> Vf/1
  GTO Logic/1(status) -> G_D/2, Diode Logic/3(G), "Vf "/1(status_GTO)
  Data Type  Conversion3/1 -> Product/1
  g/1 -> Data Type  Conversion4/1
  Data Type  Conversion4/1 -> Tail discrete/2(switch), GTO Logic/2(G)
  Diode Logic/1(status) -> Data Type  Conversion5/1
  Data Type  Conversion5/1 -> G_D/1
  Unit Delay3/1 -> status/1
  G_D/1 -> Data Type  Conversion2/1
  Data Type  Conversion2/1 -> Unit Delay3/1

== system powerlib_models/Discrete/HTG ==
  wref : Inport  Port=1  LatchInput=off
  Pref : Inport  Port=2  LatchInput=off
  we : Inport  Port=3  LatchInput=off
  Pe : Inport  Port=4  LatchInput=off
  dw : Inport  Port=5  LatchInput=off
  Constant1 : Constant  Orientation=left  Value=dref
  Discrete PID Controller : Subsystem  AncestorBlock=|  mask(Discrete PID Controller){Kp=kp, Ki=ki, Kd=kd, TcD=td, Par_Limits=[1e6 -1e6], Init=go, Ts=Ts}
      | powerlib_extras/Discrete 
      | Control Blocks/Discrete
      | PID Controller
      mask prompts: Kp "Proportional gain (Kp):"; Ki "Integral gain (Ki):"; Kd "Derivative gain (Kd):"; TcD "Time constant for derivative (s):"; Par_Limits "Output limits: [ Upper   Lower ]"; Init "Output initial value:"; Ts "Sample time:"
      mask help: This block implements a discrete PID controller.
      mask init:
      | UpperLimit=Par_Limits(1);
      | LowerLimit=Par_Limits(2);
      mask Display: disp('PID');
  Sum : Sum  Inputs=+-  SaturateOnIntegerOverflow=on  InputSameDT=on
  Sum1 : Sum  Inputs=+-  SaturateOnIntegerOverflow=on  InputSameDT=on
  Sum5 : Sum  Inputs=-+  SaturateOnIntegerOverflow=on  InputSameDT=on
  Switch : Switch  Orientation=left  Threshold=0.5  InputSameDT=on
  permanent droop : Gain  Orientation=left  Gain=Rp  SaturateOnIntegerOverflow=on
  servo-motor : Subsystem
      mask Display: disp('servo-\nmotor')
  turbine : Subsystem
      mask Display: disp('hydraulic\nturbine')
  Pm : Outport  InitialOutput=0
  gate : Outport  Port=2  InitialOutput=0
  wires:
  Constant1/1 -> Switch/2
  Switch/1 -> permanent droop/1
  Pe/1 -> Sum5/2
  Pref/1 -> Sum5/1
  Sum1/1 -> Discrete PID Controller/1(Error)
  permanent droop/1 -> Sum1/2
  Sum/1 -> Sum1/1
  Discrete PID Controller/1(Out) -> servo-motor/1(regulator's output)
  wref/1 -> Sum/1
  we/1 -> Sum/2
  Sum5/1 -> Switch/3
  servo-motor/1(gate opening) -> turbine/2(gate opening), gate/1, Switch/1
  dw/1 -> turbine/1(dw)
  turbine/1(Pm) -> Pm/1

== system powerlib_models/Discrete/Impedance Measurement ==
  v : Inport  Port=1  LatchInput=off
  Ground : Ground
  Terminator : Terminator
  i : Outport  InitialOutput=0
  wires:
  v/1 -> Terminator/1
  Ground/1 -> i/1

== system powerlib_models/Discrete/MBPSS ==
  note: (for simplified
      | settings only)
  note: Low and intermediate speed deviation is based on the internal voltage phasors while
      | the high frequency speed deviation  is based on the electrical power.
  note: Note: Speed deviation is derived from the machine positive-sequence terminal voltages and currents.
  note: (IEEE Type PSS4b)
  note: Discrete Multi-band Power System Stabilizer
  note: Innocent Kamwa, Robert Grondin
      | IREQ, Hydro-Quebec
  dw : Inport  Port=1  LatchInput=off
  Constant : Constant  Value=Detailed
  Discrete Lead-Lag1 : Subsystem  mask(Discrete Lead-Lag Compensator){values=[TL1 TL2 KL11], Ts=Ts}
      mask prompts: values "Coefficients values: [ T1 T2 K1 ]"; Ts "Sample time (s):"
      mask help:
      | This block implements a discrete lead-lag compensator:
      |
      |          T1.s + K1
      | H(s)= --------
      |            T2.s + 1
      mask init:
      | numc=[values(1) values(3)];
      | denc=[values(2) 1];
      | [Ac,Bc,Cc,Dc]=tf2ss(numc,denc);
      | %
      | %  Conversion to discrete transfer function
      | nstates = size(Ac,1);
      | invexp = inv(eye(nstates) - (Ts/2)*Ac);
      | Ad = invexp*(eye(nstates) + (Ts/2)*Ac);
      | Bd = invexp*Bc;
      | Cd = Cc*invexp*Ts;
      | Dd = Cc*invexp*Bc*(Ts/2) + Dc;
      | %
      | if values(1)==0 & values(2)==0, Dd=1; end
      mask Display: disp('TL1.s+KL11\n---\nTL2.s+1')
  Discrete Lead-Lag2 : Subsystem  mask(Discrete Lead-Lag Compensator){values=[TL7 TL8 KL17], Ts=Ts}
      mask prompts: values "Coefficients values: [ T1 T2 K1 ]"; Ts "Sample time (s):"
      mask help:
      | This block implements a discrete lead-lag compensator:
      |
      |          T1.s + K1
      | H(s)= --------
      |            T2.s + 1
      mask init: same as powerlib_models/Discrete/MBPSS/Discrete Lead-Lag1
      mask Display: disp('TL7.s+KL17\n---\nTL8.s+1')
  Discrete Lead-Lag3 : Subsystem  mask(Discrete Lead-Lag Compensator){values=[TI1 TI2 KI11], Ts=Ts}
      mask prompts: values "Coefficients values: [ T1 T2 K1 ]"; Ts "Sample time (s):"
      mask help:
      | This block implements a discrete lead-lag compensator:
      |
      |          T1.s + K1
      | H(s)= --------
      |            T2.s + 1
      mask init: same as powerlib_models/Discrete/MBPSS/Discrete Lead-Lag1
      mask Display: disp('TI1.s+KI11\n---\nTI2.s+1')
  Discrete Lead-Lag4 : Subsystem  mask(Discrete Lead-Lag Compensator){values=[TI7 TI8 KI17], Ts=Ts}
      mask prompts: values "Coefficients values: [ T1 T2 K1 ]"; Ts "Sample time (s):"
      mask help:
      | This block implements a discrete lead-lag compensator:
      |
      |          T1.s + K1
      | H(s)= --------
      |            T2.s + 1
      mask init: same as powerlib_models/Discrete/MBPSS/Discrete Lead-Lag1
      mask Display: disp('TI7.s+KI17\n---\nTI8.s+1')
  Discrete Lead-Lag5 : Subsystem  mask(Discrete Lead-Lag Compensator){values=[TH1 TH2 KH11], Ts=Ts}
      mask prompts: values "Coefficients values: [ T1 T2 K1 ]"; Ts "Sample time (s):"
      mask help:
      | This block implements a discrete lead-lag compensator:
      |
      |          T1.s + K1
      | H(s)= --------
      |            T2.s + 1
      mask init: same as powerlib_models/Discrete/MBPSS/Discrete Lead-Lag1
      mask Display: disp('TH1.s+KH11\n---\nTH2.s+1')
  Discrete Lead-Lag6 : Subsystem  mask(Discrete Lead-Lag Compensator){values=[TH7 TH8 KH17], Ts=Ts}
      mask prompts: values "Coefficients values: [ T1 T2 K1 ]"; Ts "Sample time (s):"
      mask help:
      | This block implements a discrete lead-lag compensator:
      |
      |          T1.s + K1
      | H(s)= --------
      |            T2.s + 1
      mask init: same as powerlib_models/Discrete/MBPSS/Discrete Lead-Lag1
      mask Display: disp('TH7.s+KH17\n---\nTH8.s+1')
  Gain : Gain  Gain=KL  SaturateOnIntegerOverflow=on
  Gain1 : Gain  Gain=KI  SaturateOnIntegerOverflow=on
  Gain2 : Gain  Gain=KH  SaturateOnIntegerOverflow=on
  Gain3 : Gain  Gain=KL1  SaturateOnIntegerOverflow=on
  Gain4 : Gain  Gain=KL2  SaturateOnIntegerOverflow=on
  Gain5 : Gain  Gain=KI1  SaturateOnIntegerOverflow=on
  Gain6 : Gain  Gain=KI2  SaturateOnIntegerOverflow=on
  Gain7 : Gain  Gain=KH1  SaturateOnIntegerOverflow=on
  Gain8 : Gain  Gain=KH2  SaturateOnIntegerOverflow=on
  Gain9 : Gain  Gain=Kg  SaturateOnIntegerOverflow=on
  HF speed sensor : Subsystem  mask(discrete state-space model (PSB)){numc=[80 0 0], denc=[1 82 161 80], Ts=Ts}
      mask prompts: numc "Numerator:"; denc "Denominator:"; Ts "Sample time (s):"
      mask help: This block implements a discrete state-space model based on the coefficients of a continuous transfer function. Coefficients must be given in descending power of s.
      mask init:
      | [Ac,Bc,Cc,Dc]=tf2ss(numc,denc);
      | %
      | %  Conversion to discrete transfer function
      | nstates = size(Ac,1);
      | invexp = inv(eye(nstates) - (Ts/2)*Ac);
      | Ad = invexp*(eye(nstates) + (Ts/2)*Ac);
      | Bd = invexp*Bc;
      | Cd = Cc*invexp*Ts;
      | Dd = Cc*invexp*Bc*(Ts/2) + Dc;
      mask Display: disp('Discrete\nState-space\nModel')
  LF and IF speed sensor : Subsystem  mask(discrete state-space model (PSB)){numc=[-1.759e-3 1], denc=[1.2739e-4 1.7823e-2 1], Ts=Ts}
      mask prompts: numc "Numerator:"; denc "Denominator:"; Ts "Sample time (s):"
      mask help: This block implements a discrete state-space model based on the coefficients of a continuous transfer function. Coefficients must be given in descending power of s.
      mask init: same as powerlib_models/Discrete/MBPSS/HF speed sensor
      mask Display: disp('Discrete\nState-space\nModel')
  "Limiteur BF " : Saturate  UpperLimit=LIM_VL  LowerLimit=-LIM_VL
  Limiteur HF : Saturate  UpperLimit=LIM_VH  LowerLimit=-LIM_VH
  "Limiteur IF " : Saturate  UpperLimit=LIM_VI  LowerLimit=-LIM_VI
  Limiteur VS : Saturate  UpperLimit=LIM_VS  LowerLimit=-LIM_VS
  Sum : Sum  Inputs=+-  SaturateOnIntegerOverflow=on  InputSameDT=on
  Sum1 : Sum  Inputs=+++  SaturateOnIntegerOverflow=on  InputSameDT=on
  Sum2 : Sum  Inputs=+-  SaturateOnIntegerOverflow=on  InputSameDT=on
  Sum3 : Sum  Inputs=+-  SaturateOnIntegerOverflow=on  InputSameDT=on
  Transfer function for detailed model (HF) : Subsystem
  Transfer function for detailed model (IF) : Subsystem
  Transfer function for detailed model (LF) : Subsystem
  VS : Outport  InitialOutput=0
  wires:
  Gain9/1 -> Limiteur VS/1
  Constant/1 -> Transfer function for detailed model (HF)/1(On), Transfer function for detailed model (IF)/1(On), Transfer function for detailed model (LF)/1(On)
  Limiteur VS/1 -> VS/1
  Sum1/1 -> Gain9/1
  Limiteur HF/1 -> Sum1/3
  "Limiteur IF "/1 -> Sum1/2
  "Limiteur BF "/1 -> Sum1/1
  Sum3/1 -> Gain2/1
  Transfer function for detailed model (HF)/2(LFneg) -> Sum3/2
  Transfer function for detailed model (HF)/1(HFpos) -> Sum3/1
  Discrete Lead-Lag6/1(Out1) -> Transfer function for detailed model (HF)/3("HFneg ")
  Discrete Lead-Lag5/1(Out1) -> Transfer function for detailed model (HF)/2("HFpos ")
  Sum2/1 -> Gain1/1
  Discrete Lead-Lag4/1(Out1) -> Transfer function for detailed model (IF)/3("IFneg ")
  Discrete Lead-Lag3/1(Out1) -> Transfer function for detailed model (IF)/2("IFpos ")
  Transfer function for detailed model (IF)/2(IFneg) -> Sum2/2
  Transfer function for detailed model (IF)/1(IFpos) -> Sum2/1
  Discrete Lead-Lag2/1(Out1) -> Transfer function for detailed model (LF)/3("LFneg ")
  Discrete Lead-Lag1/1(Out1) -> Transfer function for detailed model (LF)/2("LFpos ")
  Transfer function for detailed model (LF)/2(LFneg) -> Sum/2
  Transfer function for detailed model (LF)/1(LFpos) -> Sum/1
  Sum/1 -> Gain/1
  Gain/1 -> "Limiteur BF "/1
  Gain1/1 -> "Limiteur IF "/1
  Gain2/1 -> Limiteur HF/1
  Gain3/1 -> Discrete Lead-Lag1/1(In1)
  Gain4/1 -> Discrete Lead-Lag2/1(In1)
  Gain5/1 -> Discrete Lead-Lag3/1(In1)
  Gain6/1 -> Discrete Lead-Lag4/1(In1)
  Gain7/1 -> Discrete Lead-Lag5/1(In1)
  Gain8/1 -> Discrete Lead-Lag6/1(In1)
  LF and IF speed sensor/1(Out) -> Gain3/1, Gain4/1, Gain5/1, Gain6/1
  HF speed sensor/1(Out) -> Gain8/1, Gain7/1
  dw/1 -> HF speed sensor/1(In), LF and IF speed sensor/1(In)

== system powerlib_models/Discrete/PMSM_mechanics ==
  Tm : Inport  Port=1  LatchInput=off
  Te : Inport  Port=2  LatchInput=off
  Discrete-Time Integrator : DiscreteIntegrator  SampleTime=Ts  ICPrevOutput=DiscIntNeverNeededParam  ICPrevScaledInput=DiscIntNeverNeededParam
  Discrete-Time Integrator1 : DiscreteIntegrator  SampleTime=Ts  ICPrevOutput=DiscIntNeverNeededParam  ICPrevScaledInput=DiscIntNeverNeededParam
  Gain : Gain  Gain=p  SaturateOnIntegerOverflow=on
  Gain1 : Gain  Gain=1/p  SaturateOnIntegerOverflow=on
  Gain2 : Gain  Gain=1/J  SaturateOnIntegerOverflow=on
  Gain3 : Gain  Gain=F  SaturateOnIntegerOverflow=on
  Mux1 : Mux  Inputs=3
  Sum : Sum  Inputs=-+-  SaturateOnIntegerOverflow=on  InputSameDT=on
  we : Outport  InitialOutput=0
  the : Outport  Port=2  InitialOutput=0
  m : Outport  Port=3  InitialOutput=0
  wires:
  Gain3/1 -> Sum/3
  Mux1/1 -> m/1
  Tm/1 -> Sum/1
  Sum/1 -> Gain2/1
  Gain2/1 -> Discrete-Time Integrator/1
  Discrete-Time Integrator/1 -> Gain/1, Gain3/1, Mux1/1
  Gain/1 -> Discrete-Time Integrator1/1, we/1
  Te/1 -> Sum/2, Mux1/3
  Gain1/1 -> Mux1/2
  Discrete-Time Integrator1/1 -> the/1, Gain1/1

== system powerlib_models/Discrete/PM_synchronous_machine ==
  v : Inport  Port=1  LatchInput=off
  we : Inport  Port=2  LatchInput=off
  the : Inport  Port=3  LatchInput=off
  Mux : Mux  Inputs=[3,2,2]
  Selector : Selector  Elements=1:2  InputPortWidth=3
  "Te " : Fcn  Expr=1.5*p*(Flux*u(1)+(Ld-Lq)*u(1)*u(2))
  abc2qd : Subsystem
  iq,id : Subsystem
  qd2abc : Subsystem
  i : Outport  InitialOutput=0
  m : Outport  Port=2  InitialOutput=0
  Te : Outport  Port=3  InitialOutput=0
  wires:
  the/1 -> abc2qd/2(the)
  we/1 -> iq,id/2(we)
  Mux/1 -> m/1
  abc2qd/2(vq,vd) -> Mux/3, iq,id/1(vq,vd)  "vqd"
  abc2qd/1(s,c) -> qd2abc/1(s,c)
  v/1 -> abc2qd/1(Vab,Vbc)
  iq,id/1(iq,id) -> qd2abc/2(iq,id), Mux/2, "Te "/1  "iqd"
  qd2abc/1(is) -> Mux/1, Selector/1  "isabc"
  Selector/1 -> i/1
  "Te "/1 -> Te/1
